simulink model "ex1_3"  (R2024b)
settings: Solver=VariableStepAuto  StartTime=0.0  StopTime=120  RelTol=1e-3
settings Model: Creator=ceylin  LastModifiedBy=ceylin

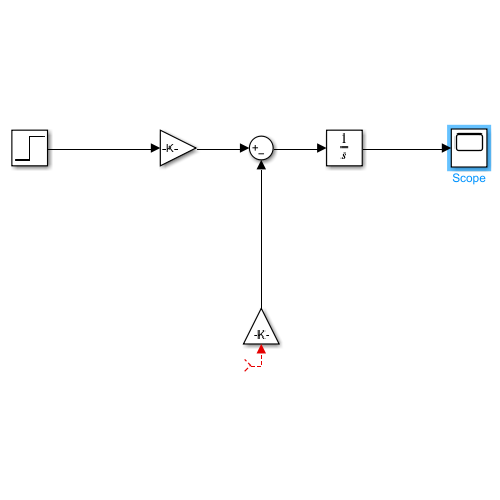
[thumbnail: Simulink's stored preview of the top-level diagram]
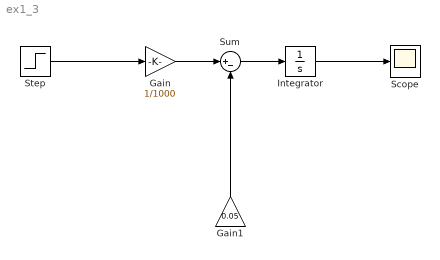
== system ex1_3 ==
  Gain : Gain  Gain=1/1000
  Gain1 : Gain  Gain=0.05
  Integrator : Integrator
  Scope : Scope
  Step : Step  Time=0  After=500  SampleTime=0
  Sum : Sum  Inputs=|+-
  wires:
  Step/1 -> Gain/1
  Gain/1 -> Sum/1
  Sum/1 -> Integrator/1
  Integrator/1 -> Scope/1
  Gain1/1 -> Sum/2
  ? -> Gain1/1
